simulink model "defilter"  (R2020b)
settings: Solver=VariableStepAuto  StartTime=0.0  StopTime=10.0  RelTol=1e-3
settings Model: Creator=com  LastModifiedBy=com

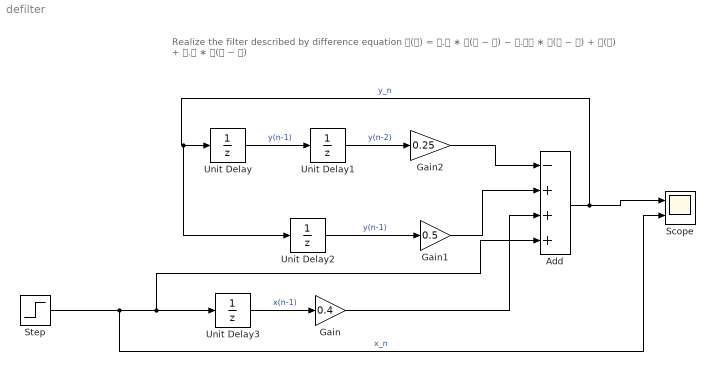
== system defilter ==
  note: Realize the filter described by difference equation 𝐲(𝐧) = 𝟎.𝟓 ∗ 𝐲(𝐧 − 𝟏) − 𝟎.𝟐𝟓 ∗ 𝐲(𝐧 − 𝟐) + 𝐱(𝐧) + 𝟎.𝟒 ∗ 𝐱(𝐧 − 𝟏)
  Add : Sum  Inputs=-+++
  Gain : Gain  Gain=0.4
  Gain1 : Gain  Gain=0.5
  Gain2 : Gain  Gain=0.25
  Scope : Scope  NumInputPorts=2
  Step : Step  SampleTime=0
  Unit Delay{,1..3} (4 alike) : UnitDelay  SampleTime=-1  HasFrameUpgradeWarning=on
  wires:
  Unit Delay/1 -> Unit Delay1/1  "y(n-1)"
  Unit Delay1/1 -> Gain2/1  "y(n-2)"
  Unit Delay3/1 -> Gain/1  "x(n-1)"
  Step/1 -> Scope/2, Add/4, Unit Delay3/1  "x_n"
  Gain2/1 -> Add/1
  Gain1/1 -> Add/2
  Add/1 -> Unit Delay2/1, Unit Delay/1, Scope/1  "y_n"
  Gain/1 -> Add/3
  Unit Delay2/1 -> Gain1/1  "y(n-1)"
